simulink model "TrackerSingleObjectCustom"  (R2023a)
settings: Solver=FixedStepDiscrete  StartTime=0.0  StopTime=inf  RelTol=1e-3  EnableMultiTasking=on
undefined symbols (not defined in the file): f
libraries: instrumentlib x1
settings Model: Creator=Ssubrama  LastModifiedBy=fedeoli
settings SolverCC: AlgebraicLoopSolver=TrustRegion
settings DataIOCC: LimitDataPoints=on  SaveFormat=Array  SignalLoggingSaveFormat=ModelDataLogs  ReturnWorkspaceOutputs=off
settings OptimizationCC: ExpressionDepthLimit=2147483647  InitFltsAndDblsToZero=on  LifeSpan=inf
settings DebuggingCC: UnderspecifiedInitializationDetection=Classic  MergeDetectMultiDrivingBlocksExec=none  SolverPrmCheckMsg=warning  FcnCallInpInsideContextMsg=warning  UnconnectedInputMsg=warning  UnconnectedOutputMsg=warning  UnconnectedLineMsg=warning  StateNameClashWarn=warning  SFUnexpectedBacktrackingDiag=warning  SFNoUnconditionalDefaultTransitionDiag=warning  SFExecutionAtInitializationDiag=none  ArithmeticOperatorsInVariantConditions=warning
settings HardwareCC: ProdBitPerPointer=32  ProdBitPerSizeT=32  ProdBitPerPtrDiffT=32  ProdLargestAtomicFloat=None  ProdIntDivRoundTo=Undefined  ProdEndianess=Unspecified  ProdWordSize=32  ProdHWDeviceType=32-bit Generic
settings ModelReferenceCC: PropagateSignalLabelsOutOfModel=off
settings SFSimCC: SimUseLocalCustomCode=off  CustomCodeUndefinedFunction=UseInterfaceOnly
settings RTWCC: RTWUseLocalCustomCode=off
settings CodeAppCC: StateflowObjectComments=on
settings GRTTargetCC: TargetFcnLib=ansi_tfl_tmw_new.mat  TargetLangStandard=C89/C90 (ANSI)  CombineOutputUpdateFcns=off  GRTInterface=on
settings ConfigComp: CovMetricSettings=dw  CovSaveCumulativeToWorkspaceVar=on  CovSaveSingleToWorkspaceVar=on  CovExternalEMLEnable=off  CovSFcnEnable=off

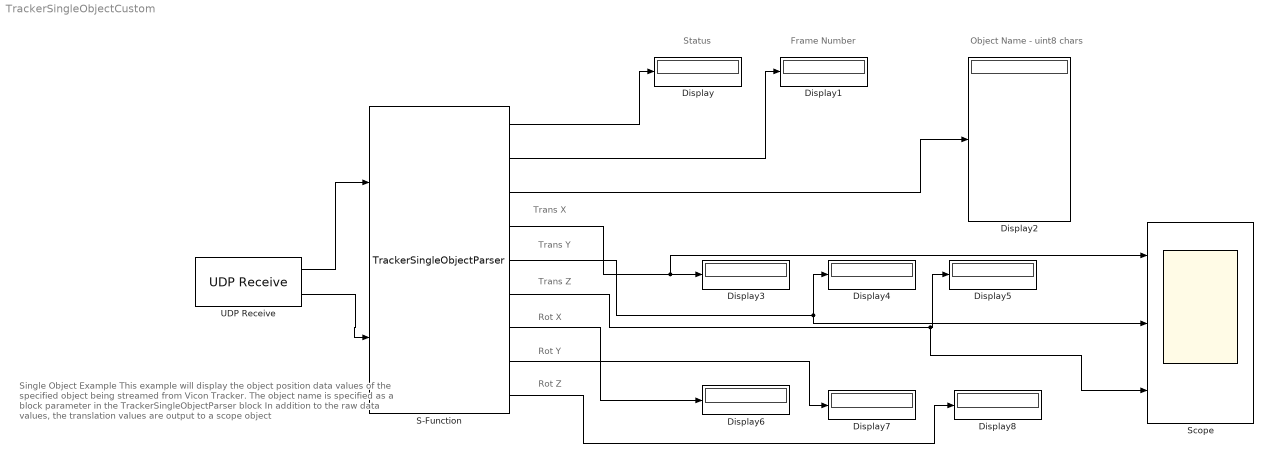
== system TrackerSingleObjectCustom ==
  note: Rot Z
  note: Rot Y
  note: Rot X
  note: Trans Z
  note: Trans Y
  note: Trans X
  note: Single Object Example
      |
      | This example will display the object position data
      | values of the specified object being streamed from
      | Vicon Tracker.
      |
      | The object name is specified as a block parameter
      | in the TrackerSingleObjectParser block
      |
      | In addition to the raw data values, the
      | translation values are output to a scope object
  note: Object Name - uint8 chars
  note: Frame Number
  note: Status
  Display{,1..8} (9 alike) : Display
  S-Function : S-Function  FunctionName=TrackerSingleObjectParser  Parameters='chen'  SFunctionModules=TrackerSingleObjectParser  SFunctionDeploymentMode=off  EnableBusSupport=off
      settings: AttributesFormatString=Data Parser
  Scope : Scope  NumInputPorts=3
  UDP Receive : instrumentlib/UDP Receive  Priority=3  LocalAddress=0.0.0.0  LocalPort=51001  EnablePortSharing=off  Host=132.68.134.248  Port=801  GetLatestData=off  DataSize=256  DataType=uint8  ASCIIFormatting=%f,  Terminator=LF  CustomTerminator=10  ByteOrder=big-endian  EnableBlockingMode=off  Timeout=inf  SampleTime=0.01  SimulateUsing=Interpreted execution
  wires:
  UDP Receive/1 -> S-Function/1
  S-Function/1 -> Display/1
  UDP Receive/2 -> S-Function/2
  S-Function/2 -> Display1/1
  S-Function/3 -> Display2/1
  S-Function/5 -> Display4/1, Scope/2
  S-Function/6 -> Scope/3, Display5/1
  S-Function/7 -> Display6/1
  S-Function/8 -> Display7/1
  S-Function/9 -> Display8/1
  S-Function/4 -> Scope/1, Display3/1
